simulink model "week8_trial"  (R2020b)
settings: Solver=VariableStepAuto  StartTime=0.0  StopTime=100  FixedStep=0.1  RelTol=1e-3
undefined symbols (not defined in the file or in its folder): Cf, Cr, Iz, lf, lr, m, md, sigbuilder_block, Ts, V_init
libraries: pid_lib x2, mpcadaslib x1
(part 2 of 2)

== matlab function week8_trial/Sensor data /Lateral control sensor inputs/Subsystem/MATLAB Function ==
  settings: updateMethod=DISCRETE  sampleTime=ts
  data: data parameter; seq output; steps parameter; t input; first output; next_t output
function [seq,first,next_t] = fcn(data,steps,t)
%#codegen
[seq,first,next_t] = mpcblock_preview('md',data,steps,t);

== stateflow chart week8_trial/Adaptive Cruise control/ACC/feedforward performance/quadrant chart ==
  state quadrant2
    entry:
    quadrant  = 2;
  state quadrant1
    entry:
    quadrant  = 1;
  state quadrant4
    entry:
    quadrant  = 4;
  state quadrant3
    entry:
    quadrant  = 3;
  (default) -> quadrant1
  quadrant1 -> (junction 7) : [((R<R_c) || (v_target< v_host))&& after(10,sec)]
  (junction 7) -> quadrant2 [order 4] : [(R>R_c)&&(v_target < v_host)]
  quadrant2 -> (junction 7) : [((R>R_c) || (v_target> v_host))&& after(10,sec)]
  (junction 7) -> quadrant1 [order 1] : [(R>R_c)&&(v_target > v_host) ]
  quadrant3 -> (junction 7) : [((R>R_c) || (v_target> v_host)&& after(10,sec))]
  (junction 7) -> quadrant3 [order 3] : [(R<R_c)&&(v_target < v_host)]
  quadrant4 -> (junction 7) : [((R>R_c) || (v_target< v_host))&& after(10,sec)]
  (junction 7) -> quadrant4 [order 2] : [(R<R_c)&&(v_target > v_host) ]
  data: R_c input; v_host input; v_target input; quadrant output; R input

== stateflow chart week8_trial/Adaptive Cruise control/ACC/ACC State logic/ACC state control ==
  state HeadwayControl
    entry: en_man=false;
    en_vel = false;
    en_pos = true;
  state Manual__
    entry: en_man=true;
    en_vel = false;
    en_pos = false;
  state VelocityControl_
    entry: en_man=false ;
    en_vel = true;
    en_pos = false;
  Manual__ -> VelocityControl_ [order 1] : [(ACC_enable==1) &(target_flag==0)]
  Manual__ -> HeadwayControl [order 2] : [(ACC_enable==1) &(target_flag==1)]
  VelocityControl_ -> HeadwayControl [order 2] : [(ACC_enable==1) &(target_flag==1)&& after(10,sec) ]
  (default) -> Manual__
  VelocityControl_ -> Manual__ [order 1] : [(ACC_enable==0) ]
  HeadwayControl -> VelocityControl_ [order 2] : [((ACC_enable==1) &(target_flag==0) || V_host >commanded_speed+0.5) &&after(20,sec) ]
  HeadwayControl -> Manual__ [order 1] : [(ACC_enable==0) ]
  data: en_man output; en_pos output; en_vel output; ACC_enable input; commanded_speed input; V_host input; target_flag input

== stateflow chart week8_trial/HA mode manager/Subsystem/Chart ==
  state HA_Off
    entry: en_manual = true;
    HA_active = false
  state HA_ON
    state Hands_ON
      entry: en_manual = false;
      HA_active = true;
      Hands_on = true;
    state Hands_Off
      entry: en_manual = false;
      HA_active = true;
      Hands_on = false;
    (default) -> Hands_ON
    Hands_ON -> Hands_Off : [Hands_off_zone == 1]
    Hands_Off -> Hands_ON : [Hands_off_zone == 0]
  (default) -> HA_Off
  HA_ON -> HA_Off : [(ACC_enable == 0)||(HA_available==0)||(LCA_enable==0)]
  HA_Off -> HA_ON : [(ACC_enable == 1)&&(HA_available==1)&&(LCA_enable==1)]
  data: ACC_enable input; HA_available input; LCA_enable input; HA_active output; Hands_on output; en_manual output; Hands_off_zone input
